simulink model "dft_8_point"  (R2016b)
settings: Solver=VariableStepDiscrete  StartTime=0.0  StopTime=12/fs  RelTol=1e-3  EnableMultiTasking=on
PreLoadFcn:
  | t = 2;
  | b = 14;
  | 
  | fs = 1;
StartFcn:
  | close all;
StopFcn:
  | % create matrices of Re and Im parts over time - inputs
  | xin_re = [xin_0_re xin_1_re xin_2_re xin_3_re xin_4_re xin_5_re xin_6_re xin_7_re];
  | xin_im = [xin_0_im xin_0_im xin_0_im xin_0_im xin_0_im xin_0_im xin_0_im xin_0_im];
  | 
  | % create matrices of Re and Im parts over time - outputs
  | X_re = [X0_re X1_re X2_re X3_re X4_re X5_re X6_re X7_re];
  | X_im = [X0_im X1_im X2_im X3_im X4_im X5_im X6_im X7_im];
  | 
  | % create vectors of Magnitudes and Angles over time
  | X_mag = [X0_mag X1_mag X2_mag X3_mag X4_mag X5_mag X6_mag X7_mag];
  | X_ang = [X0_ang X1_ang X2_ang X3_ang X4_ang X5_ang X6_ang X7_ang];
  | 
  | 
  | figure(1)
  | hold off
  | plot([0:1:7],xin_re(end,:),'r-o','MarkerFaceColor','r');
  | hold on
  | plot([0:1:7],xin_im(end,:),'b-o','MarkerFaceColor','b');
  | xlabel('Samples');
  | ylabel('Magnitude');
  | title('Input to DFT');
  | legend('Real','Imaginary','Location','EastOutside')
  | grid on;
  | 
  | set(1,'Name','Input to DFT','NumberTitle','off');
  | % setStandardFigSize(1);
  | 
  | figure(2)
  | hold off
  | plot([0:1:7],X_mag(end,:),'k-o','MarkerFaceColor','b');
  | hold on
  | xlabel('Frequency Bin');
  | ylabel('Magnitude');
  | grid on;
  | title('Magnitude DFT Plot');
  | 
  | set(2,'Name','Output of DFT','NumberTitle','off');
  | % setStandardFigSize(2);
libraries: xbsIndex_r4 x955
(part 8 of 8)

== system dft_8_point/cplx_add45 ==
  a_im : Inport
  b_im : Inport  Port=2
  a_re : Inport  Port=3
  b_re : Inport  Port=4
  AddSub13 : xbsIndex_r4/AddSub  mode=Addition  use_carryin=off  use_carryout=off  en=off  latency=0  precision=User Defined  arith_type="Signed  (2's comp)"  n_bits=t+b  bin_pt=b  quantization=Truncate  overflow=Wrap  use_behavioral_HDL=off  hw_selection=Fabric  pipelined=off  dbl_ovrd=off  block_type=addsub
  AddSub6 : xbsIndex_r4/AddSub  mode=Addition  use_carryin=off  use_carryout=off  en=off  latency=0  precision=User Defined  arith_type="Signed  (2's comp)"  n_bits=t+b  bin_pt=b  quantization=Truncate  overflow=Wrap  use_behavioral_HDL=off  hw_selection=Fabric  pipelined=off  dbl_ovrd=off  block_type=addsub
  im : Outport
  re : Outport  Port=2
  wires:
  a_im/1 -> AddSub6/1
  AddSub6/1 -> im/1
  b_im/1 -> AddSub6/2
  a_re/1 -> AddSub13/1
  AddSub13/1 -> re/1
  b_re/1 -> AddSub13/2

== system dft_8_point/cplx_add46 ==
  a_im : Inport
  b_im : Inport  Port=2
  a_re : Inport  Port=3
  b_re : Inport  Port=4
  AddSub13 : xbsIndex_r4/AddSub  mode=Addition  use_carryin=off  use_carryout=off  en=off  latency=0  precision=User Defined  arith_type="Signed  (2's comp)"  n_bits=t+b  bin_pt=b  quantization=Truncate  overflow=Wrap  use_behavioral_HDL=off  hw_selection=Fabric  pipelined=off  dbl_ovrd=off  block_type=addsub
  AddSub6 : xbsIndex_r4/AddSub  mode=Addition  use_carryin=off  use_carryout=off  en=off  latency=0  precision=User Defined  arith_type="Signed  (2's comp)"  n_bits=t+b  bin_pt=b  quantization=Truncate  overflow=Wrap  use_behavioral_HDL=off  hw_selection=Fabric  pipelined=off  dbl_ovrd=off  block_type=addsub
  im : Outport
  re : Outport  Port=2
  wires:
  a_im/1 -> AddSub6/1
  AddSub6/1 -> im/1
  b_im/1 -> AddSub6/2
  a_re/1 -> AddSub13/1
  AddSub13/1 -> re/1
  b_re/1 -> AddSub13/2

== system dft_8_point/cplx_add47 ==
  a_im : Inport
  b_im : Inport  Port=2
  a_re : Inport  Port=3
  b_re : Inport  Port=4
  AddSub13 : xbsIndex_r4/AddSub  mode=Addition  use_carryin=off  use_carryout=off  en=off  latency=0  precision=User Defined  arith_type="Signed  (2's comp)"  n_bits=t+b  bin_pt=b  quantization=Truncate  overflow=Wrap  use_behavioral_HDL=off  hw_selection=Fabric  pipelined=off  dbl_ovrd=off  block_type=addsub
  AddSub6 : xbsIndex_r4/AddSub  mode=Addition  use_carryin=off  use_carryout=off  en=off  latency=0  precision=User Defined  arith_type="Signed  (2's comp)"  n_bits=t+b  bin_pt=b  quantization=Truncate  overflow=Wrap  use_behavioral_HDL=off  hw_selection=Fabric  pipelined=off  dbl_ovrd=off  block_type=addsub
  im : Outport
  re : Outport  Port=2
  wires:
  a_im/1 -> AddSub6/1
  AddSub6/1 -> im/1
  b_im/1 -> AddSub6/2
  a_re/1 -> AddSub13/1
  AddSub13/1 -> re/1
  b_re/1 -> AddSub13/2

== system dft_8_point/cplx_add48 ==
  a_im : Inport
  b_im : Inport  Port=2
  a_re : Inport  Port=3
  b_re : Inport  Port=4
  AddSub13 : xbsIndex_r4/AddSub  mode=Addition  use_carryin=off  use_carryout=off  en=off  latency=0  precision=User Defined  arith_type="Signed  (2's comp)"  n_bits=t+b  bin_pt=b  quantization=Truncate  overflow=Wrap  use_behavioral_HDL=off  hw_selection=Fabric  pipelined=off  dbl_ovrd=off  block_type=addsub
  AddSub6 : xbsIndex_r4/AddSub  mode=Addition  use_carryin=off  use_carryout=off  en=off  latency=0  precision=User Defined  arith_type="Signed  (2's comp)"  n_bits=t+b  bin_pt=b  quantization=Truncate  overflow=Wrap  use_behavioral_HDL=off  hw_selection=Fabric  pipelined=off  dbl_ovrd=off  block_type=addsub
  im : Outport
  re : Outport  Port=2
  wires:
  a_im/1 -> AddSub6/1
  AddSub6/1 -> im/1
  b_im/1 -> AddSub6/2
  a_re/1 -> AddSub13/1
  AddSub13/1 -> re/1
  b_re/1 -> AddSub13/2

== system dft_8_point/cplx_add49 ==
  a_im : Inport
  b_im : Inport  Port=2
  a_re : Inport  Port=3
  b_re : Inport  Port=4
  AddSub13 : xbsIndex_r4/AddSub  mode=Addition  use_carryin=off  use_carryout=off  en=off  latency=0  precision=User Defined  arith_type="Signed  (2's comp)"  n_bits=t+b  bin_pt=b  quantization=Truncate  overflow=Wrap  use_behavioral_HDL=off  hw_selection=Fabric  pipelined=off  dbl_ovrd=off  block_type=addsub
  AddSub6 : xbsIndex_r4/AddSub  mode=Addition  use_carryin=off  use_carryout=off  en=off  latency=0  precision=User Defined  arith_type="Signed  (2's comp)"  n_bits=t+b  bin_pt=b  quantization=Truncate  overflow=Wrap  use_behavioral_HDL=off  hw_selection=Fabric  pipelined=off  dbl_ovrd=off  block_type=addsub
  im : Outport
  re : Outport  Port=2
  wires:
  a_im/1 -> AddSub6/1
  AddSub6/1 -> im/1
  b_im/1 -> AddSub6/2
  a_re/1 -> AddSub13/1
  AddSub13/1 -> re/1
  b_re/1 -> AddSub13/2

== system dft_8_point/cplx_add5 ==
  a_im : Inport
  b_im : Inport  Port=2
  a_re : Inport  Port=3
  b_re : Inport  Port=4
  AddSub13 : xbsIndex_r4/AddSub  mode=Addition  use_carryin=off  use_carryout=off  en=off  latency=0  precision=User Defined  arith_type="Signed  (2's comp)"  n_bits=t+b  bin_pt=b  quantization=Truncate  overflow=Wrap  use_behavioral_HDL=off  hw_selection=Fabric  pipelined=off  dbl_ovrd=off  block_type=addsub
  AddSub6 : xbsIndex_r4/AddSub  mode=Addition  use_carryin=off  use_carryout=off  en=off  latency=0  precision=User Defined  arith_type="Signed  (2's comp)"  n_bits=t+b  bin_pt=b  quantization=Truncate  overflow=Wrap  use_behavioral_HDL=off  hw_selection=Fabric  pipelined=off  dbl_ovrd=off  block_type=addsub
  im : Outport
  re : Outport  Port=2
  wires:
  a_im/1 -> AddSub6/1
  AddSub6/1 -> im/1
  b_im/1 -> AddSub6/2
  a_re/1 -> AddSub13/1
  AddSub13/1 -> re/1
  b_re/1 -> AddSub13/2

== system dft_8_point/cplx_add50 ==
  a_im : Inport
  b_im : Inport  Port=2
  a_re : Inport  Port=3
  b_re : Inport  Port=4
  AddSub13 : xbsIndex_r4/AddSub  mode=Addition  use_carryin=off  use_carryout=off  en=off  latency=0  precision=User Defined  arith_type="Signed  (2's comp)"  n_bits=t+b  bin_pt=b  quantization=Truncate  overflow=Wrap  use_behavioral_HDL=off  hw_selection=Fabric  pipelined=off  dbl_ovrd=off  block_type=addsub
  AddSub6 : xbsIndex_r4/AddSub  mode=Addition  use_carryin=off  use_carryout=off  en=off  latency=0  precision=User Defined  arith_type="Signed  (2's comp)"  n_bits=t+b  bin_pt=b  quantization=Truncate  overflow=Wrap  use_behavioral_HDL=off  hw_selection=Fabric  pipelined=off  dbl_ovrd=off  block_type=addsub
  im : Outport
  re : Outport  Port=2
  wires:
  a_im/1 -> AddSub6/1
  AddSub6/1 -> im/1
  b_im/1 -> AddSub6/2
  a_re/1 -> AddSub13/1
  AddSub13/1 -> re/1
  b_re/1 -> AddSub13/2

== system dft_8_point/cplx_add51 ==
  a_im : Inport
  b_im : Inport  Port=2
  a_re : Inport  Port=3
  b_re : Inport  Port=4
  AddSub13 : xbsIndex_r4/AddSub  mode=Addition  use_carryin=off  use_carryout=off  en=off  latency=0  precision=User Defined  arith_type="Signed  (2's comp)"  n_bits=t+b  bin_pt=b  quantization=Truncate  overflow=Wrap  use_behavioral_HDL=off  hw_selection=Fabric  pipelined=off  dbl_ovrd=off  block_type=addsub
  AddSub6 : xbsIndex_r4/AddSub  mode=Addition  use_carryin=off  use_carryout=off  en=off  latency=0  precision=User Defined  arith_type="Signed  (2's comp)"  n_bits=t+b  bin_pt=b  quantization=Truncate  overflow=Wrap  use_behavioral_HDL=off  hw_selection=Fabric  pipelined=off  dbl_ovrd=off  block_type=addsub
  im : Outport
  re : Outport  Port=2
  wires:
  a_im/1 -> AddSub6/1
  AddSub6/1 -> im/1
  b_im/1 -> AddSub6/2
  a_re/1 -> AddSub13/1
  AddSub13/1 -> re/1
  b_re/1 -> AddSub13/2

== system dft_8_point/cplx_add52 ==
  a_im : Inport
  b_im : Inport  Port=2
  a_re : Inport  Port=3
  b_re : Inport  Port=4
  AddSub13 : xbsIndex_r4/AddSub  mode=Addition  use_carryin=off  use_carryout=off  en=off  latency=0  precision=User Defined  arith_type="Signed  (2's comp)"  n_bits=t+b  bin_pt=b  quantization=Truncate  overflow=Wrap  use_behavioral_HDL=off  hw_selection=Fabric  pipelined=off  dbl_ovrd=off  block_type=addsub
  AddSub6 : xbsIndex_r4/AddSub  mode=Addition  use_carryin=off  use_carryout=off  en=off  latency=0  precision=User Defined  arith_type="Signed  (2's comp)"  n_bits=t+b  bin_pt=b  quantization=Truncate  overflow=Wrap  use_behavioral_HDL=off  hw_selection=Fabric  pipelined=off  dbl_ovrd=off  block_type=addsub
  im : Outport
  re : Outport  Port=2
  wires:
  a_im/1 -> AddSub6/1
  AddSub6/1 -> im/1
  b_im/1 -> AddSub6/2
  a_re/1 -> AddSub13/1
  AddSub13/1 -> re/1
  b_re/1 -> AddSub13/2

== system dft_8_point/cplx_add53 ==
  a_im : Inport
  b_im : Inport  Port=2
  a_re : Inport  Port=3
  b_re : Inport  Port=4
  AddSub13 : xbsIndex_r4/AddSub  mode=Addition  use_carryin=off  use_carryout=off  en=off  latency=0  precision=User Defined  arith_type="Signed  (2's comp)"  n_bits=t+b  bin_pt=b  quantization=Truncate  overflow=Wrap  use_behavioral_HDL=off  hw_selection=Fabric  pipelined=off  dbl_ovrd=off  block_type=addsub
  AddSub6 : xbsIndex_r4/AddSub  mode=Addition  use_carryin=off  use_carryout=off  en=off  latency=0  precision=User Defined  arith_type="Signed  (2's comp)"  n_bits=t+b  bin_pt=b  quantization=Truncate  overflow=Wrap  use_behavioral_HDL=off  hw_selection=Fabric  pipelined=off  dbl_ovrd=off  block_type=addsub
  im : Outport
  re : Outport  Port=2
  wires:
  a_im/1 -> AddSub6/1
  AddSub6/1 -> im/1
  b_im/1 -> AddSub6/2
  a_re/1 -> AddSub13/1
  AddSub13/1 -> re/1
  b_re/1 -> AddSub13/2

== system dft_8_point/cplx_add54 ==
  a_im : Inport
  b_im : Inport  Port=2
  a_re : Inport  Port=3
  b_re : Inport  Port=4
  AddSub13 : xbsIndex_r4/AddSub  mode=Addition  use_carryin=off  use_carryout=off  en=off  latency=0  precision=User Defined  arith_type="Signed  (2's comp)"  n_bits=t+b  bin_pt=b  quantization=Truncate  overflow=Wrap  use_behavioral_HDL=off  hw_selection=Fabric  pipelined=off  dbl_ovrd=off  block_type=addsub
  AddSub6 : xbsIndex_r4/AddSub  mode=Addition  use_carryin=off  use_carryout=off  en=off  latency=0  precision=User Defined  arith_type="Signed  (2's comp)"  n_bits=t+b  bin_pt=b  quantization=Truncate  overflow=Wrap  use_behavioral_HDL=off  hw_selection=Fabric  pipelined=off  dbl_ovrd=off  block_type=addsub
  im : Outport
  re : Outport  Port=2
  wires:
  a_im/1 -> AddSub6/1
  AddSub6/1 -> im/1
  b_im/1 -> AddSub6/2
  a_re/1 -> AddSub13/1
  AddSub13/1 -> re/1
  b_re/1 -> AddSub13/2

== system dft_8_point/cplx_add55 ==
  a_im : Inport
  b_im : Inport  Port=2
  a_re : Inport  Port=3
  b_re : Inport  Port=4
  AddSub13 : xbsIndex_r4/AddSub  mode=Addition  use_carryin=off  use_carryout=off  en=off  latency=0  precision=User Defined  arith_type="Signed  (2's comp)"  n_bits=t+b  bin_pt=b  quantization=Truncate  overflow=Wrap  use_behavioral_HDL=off  hw_selection=Fabric  pipelined=off  dbl_ovrd=off  block_type=addsub
  AddSub6 : xbsIndex_r4/AddSub  mode=Addition  use_carryin=off  use_carryout=off  en=off  latency=0  precision=User Defined  arith_type="Signed  (2's comp)"  n_bits=t+b  bin_pt=b  quantization=Truncate  overflow=Wrap  use_behavioral_HDL=off  hw_selection=Fabric  pipelined=off  dbl_ovrd=off  block_type=addsub
  im : Outport
  re : Outport  Port=2
  wires:
  a_im/1 -> AddSub6/1
  AddSub6/1 -> im/1
  b_im/1 -> AddSub6/2
  a_re/1 -> AddSub13/1
  AddSub13/1 -> re/1
  b_re/1 -> AddSub13/2

== system dft_8_point/cplx_add6 ==
  a_im : Inport
  b_im : Inport  Port=2
  a_re : Inport  Port=3
  b_re : Inport  Port=4
  AddSub13 : xbsIndex_r4/AddSub  mode=Addition  use_carryin=off  use_carryout=off  en=off  latency=0  precision=User Defined  arith_type="Signed  (2's comp)"  n_bits=t+b  bin_pt=b  quantization=Truncate  overflow=Wrap  use_behavioral_HDL=off  hw_selection=Fabric  pipelined=off  dbl_ovrd=off  block_type=addsub
  AddSub6 : xbsIndex_r4/AddSub  mode=Addition  use_carryin=off  use_carryout=off  en=off  latency=0  precision=User Defined  arith_type="Signed  (2's comp)"  n_bits=t+b  bin_pt=b  quantization=Truncate  overflow=Wrap  use_behavioral_HDL=off  hw_selection=Fabric  pipelined=off  dbl_ovrd=off  block_type=addsub
  im : Outport
  re : Outport  Port=2
  wires:
  a_im/1 -> AddSub6/1
  AddSub6/1 -> im/1
  b_im/1 -> AddSub6/2
  a_re/1 -> AddSub13/1
  AddSub13/1 -> re/1
  b_re/1 -> AddSub13/2

== system dft_8_point/cplx_add7 ==
  a_im : Inport
  b_im : Inport  Port=2
  a_re : Inport  Port=3
  b_re : Inport  Port=4
  AddSub13 : xbsIndex_r4/AddSub  mode=Addition  use_carryin=off  use_carryout=off  en=off  latency=0  precision=User Defined  arith_type="Signed  (2's comp)"  n_bits=t+b  bin_pt=b  quantization=Truncate  overflow=Wrap  use_behavioral_HDL=off  hw_selection=Fabric  pipelined=off  dbl_ovrd=off  block_type=addsub
  AddSub6 : xbsIndex_r4/AddSub  mode=Addition  use_carryin=off  use_carryout=off  en=off  latency=0  precision=User Defined  arith_type="Signed  (2's comp)"  n_bits=t+b  bin_pt=b  quantization=Truncate  overflow=Wrap  use_behavioral_HDL=off  hw_selection=Fabric  pipelined=off  dbl_ovrd=off  block_type=addsub
  im : Outport
  re : Outport  Port=2
  wires:
  a_im/1 -> AddSub6/1
  AddSub6/1 -> im/1
  b_im/1 -> AddSub6/2
  a_re/1 -> AddSub13/1
  AddSub13/1 -> re/1
  b_re/1 -> AddSub13/2

== system dft_8_point/cplx_add8 ==
  a_im : Inport
  b_im : Inport  Port=2
  a_re : Inport  Port=3
  b_re : Inport  Port=4
  AddSub13 : xbsIndex_r4/AddSub  mode=Addition  use_carryin=off  use_carryout=off  en=off  latency=0  precision=User Defined  arith_type="Signed  (2's comp)"  n_bits=t+b  bin_pt=b  quantization=Truncate  overflow=Wrap  use_behavioral_HDL=off  hw_selection=Fabric  pipelined=off  dbl_ovrd=off  block_type=addsub
  AddSub6 : xbsIndex_r4/AddSub  mode=Addition  use_carryin=off  use_carryout=off  en=off  latency=0  precision=User Defined  arith_type="Signed  (2's comp)"  n_bits=t+b  bin_pt=b  quantization=Truncate  overflow=Wrap  use_behavioral_HDL=off  hw_selection=Fabric  pipelined=off  dbl_ovrd=off  block_type=addsub
  im : Outport
  re : Outport  Port=2
  wires:
  a_im/1 -> AddSub6/1
  AddSub6/1 -> im/1
  b_im/1 -> AddSub6/2
  a_re/1 -> AddSub13/1
  AddSub13/1 -> re/1
  b_re/1 -> AddSub13/2

== system dft_8_point/cplx_add9 ==
  a_im : Inport
  b_im : Inport  Port=2
  a_re : Inport  Port=3
  b_re : Inport  Port=4
  AddSub13 : xbsIndex_r4/AddSub  mode=Addition  use_carryin=off  use_carryout=off  en=off  latency=0  precision=User Defined  arith_type="Signed  (2's comp)"  n_bits=t+b  bin_pt=b  quantization=Truncate  overflow=Wrap  use_behavioral_HDL=off  hw_selection=Fabric  pipelined=off  dbl_ovrd=off  block_type=addsub
  AddSub6 : xbsIndex_r4/AddSub  mode=Addition  use_carryin=off  use_carryout=off  en=off  latency=0  precision=User Defined  arith_type="Signed  (2's comp)"  n_bits=t+b  bin_pt=b  quantization=Truncate  overflow=Wrap  use_behavioral_HDL=off  hw_selection=Fabric  pipelined=off  dbl_ovrd=off  block_type=addsub
  im : Outport
  re : Outport  Port=2
  wires:
  a_im/1 -> AddSub6/1
  AddSub6/1 -> im/1
  b_im/1 -> AddSub6/2
  a_re/1 -> AddSub13/1
  AddSub13/1 -> re/1
  b_re/1 -> AddSub13/2

== system dft_8_point/Capture Delay Line Inputs/cplx_split1 ==
  cmplx : Inport
  Reinterpret : xbsIndex_r4/Reinterpret  force_arith_type=on  arith_type="Signed  (2's comp)"  force_bin_pt=on  bin_pt=b  block_type=reinterpret
      settings: infoedit="Changes signal type without altering the binary representation.   You can changed the signal between signed and unsigned, and relocate the binary point.<br><br>Hardware notes: In hardware this block costs nothing.<br><br>Example:  Suppose the input is 6 bits wide, signed, with 2 fractional bits, and the output is forced to unsigned with 0 fractional bits.  Then an input of -2.0 (1110.00 in binary 2's complement) becomes an output of 56 (111000 in binary)."
  Reinterpret1 : xbsIndex_r4/Reinterpret  force_arith_type=on  arith_type="Signed  (2's comp)"  force_bin_pt=on  bin_pt=b  block_type=reinterpret
      settings: infoedit="Changes signal type without altering the binary representation.   You can changed the signal between signed and unsigned, and relocate the binary point.<br><br>Hardware notes: In hardware this block costs nothing.<br><br>Example:  Suppose the input is 6 bits wide, signed, with 2 fractional bits, and the output is forced to unsigned with 0 fractional bits.  Then an input of -2.0 (1110.00 in binary 2's complement) becomes an output of 56 (111000 in binary)."
  x_imaginary : xbsIndex_r4/Slice  nbits=t+b  boolean_output=off  mode=Lower Bit Location + Width  bit1=0  base1=MSB of Input  bit0=0  base0=LSB of Input  dbl_ovrd=off  block_type=slice
  x_real : xbsIndex_r4/Slice  nbits=t+b  boolean_output=off  mode=Upper Bit Location + Width  bit1=0  base1=MSB of Input  bit0=0  base0=LSB of Input  dbl_ovrd=off  block_type=slice
  real : Outport
  imag : Outport  Port=2
  wires:
  cmplx/1 -> x_real/1, x_imaginary/1
  x_real/1 -> Reinterpret/1
  x_imaginary/1 -> Reinterpret1/1
  Reinterpret/1 -> real/1
  Reinterpret1/1 -> imag/1

== system dft_8_point/Capture Delay Line Inputs/cplx_split2 ==
  cmplx : Inport
  Reinterpret : xbsIndex_r4/Reinterpret  force_arith_type=on  arith_type="Signed  (2's comp)"  force_bin_pt=on  bin_pt=b  block_type=reinterpret
      settings: infoedit="Changes signal type without altering the binary representation.   You can changed the signal between signed and unsigned, and relocate the binary point.<br><br>Hardware notes: In hardware this block costs nothing.<br><br>Example:  Suppose the input is 6 bits wide, signed, with 2 fractional bits, and the output is forced to unsigned with 0 fractional bits.  Then an input of -2.0 (1110.00 in binary 2's complement) becomes an output of 56 (111000 in binary)."
  Reinterpret1 : xbsIndex_r4/Reinterpret  force_arith_type=on  arith_type="Signed  (2's comp)"  force_bin_pt=on  bin_pt=b  block_type=reinterpret
      settings: infoedit="Changes signal type without altering the binary representation.   You can changed the signal between signed and unsigned, and relocate the binary point.<br><br>Hardware notes: In hardware this block costs nothing.<br><br>Example:  Suppose the input is 6 bits wide, signed, with 2 fractional bits, and the output is forced to unsigned with 0 fractional bits.  Then an input of -2.0 (1110.00 in binary 2's complement) becomes an output of 56 (111000 in binary)."
  x_imaginary : xbsIndex_r4/Slice  nbits=t+b  boolean_output=off  mode=Lower Bit Location + Width  bit1=0  base1=MSB of Input  bit0=0  base0=LSB of Input  dbl_ovrd=off  block_type=slice
  x_real : xbsIndex_r4/Slice  nbits=t+b  boolean_output=off  mode=Upper Bit Location + Width  bit1=0  base1=MSB of Input  bit0=0  base0=LSB of Input  dbl_ovrd=off  block_type=slice
  real : Outport
  imag : Outport  Port=2
  wires:
  cmplx/1 -> x_real/1, x_imaginary/1
  x_real/1 -> Reinterpret/1
  x_imaginary/1 -> Reinterpret1/1
  Reinterpret/1 -> real/1
  Reinterpret1/1 -> imag/1

== system dft_8_point/Capture Delay Line Inputs/cplx_split3 ==
  cmplx : Inport
  Reinterpret : xbsIndex_r4/Reinterpret  force_arith_type=on  arith_type="Signed  (2's comp)"  force_bin_pt=on  bin_pt=b  block_type=reinterpret
      settings: infoedit="Changes signal type without altering the binary representation.   You can changed the signal between signed and unsigned, and relocate the binary point.<br><br>Hardware notes: In hardware this block costs nothing.<br><br>Example:  Suppose the input is 6 bits wide, signed, with 2 fractional bits, and the output is forced to unsigned with 0 fractional bits.  Then an input of -2.0 (1110.00 in binary 2's complement) becomes an output of 56 (111000 in binary)."
  Reinterpret1 : xbsIndex_r4/Reinterpret  force_arith_type=on  arith_type="Signed  (2's comp)"  force_bin_pt=on  bin_pt=b  block_type=reinterpret
      settings: infoedit="Changes signal type without altering the binary representation.   You can changed the signal between signed and unsigned, and relocate the binary point.<br><br>Hardware notes: In hardware this block costs nothing.<br><br>Example:  Suppose the input is 6 bits wide, signed, with 2 fractional bits, and the output is forced to unsigned with 0 fractional bits.  Then an input of -2.0 (1110.00 in binary 2's complement) becomes an output of 56 (111000 in binary)."
  x_imaginary : xbsIndex_r4/Slice  nbits=t+b  boolean_output=off  mode=Lower Bit Location + Width  bit1=0  base1=MSB of Input  bit0=0  base0=LSB of Input  dbl_ovrd=off  block_type=slice
  x_real : xbsIndex_r4/Slice  nbits=t+b  boolean_output=off  mode=Upper Bit Location + Width  bit1=0  base1=MSB of Input  bit0=0  base0=LSB of Input  dbl_ovrd=off  block_type=slice
  real : Outport
  imag : Outport  Port=2
  wires:
  cmplx/1 -> x_real/1, x_imaginary/1
  x_real/1 -> Reinterpret/1
  x_imaginary/1 -> Reinterpret1/1
  Reinterpret/1 -> real/1
  Reinterpret1/1 -> imag/1

== system dft_8_point/Capture Delay Line Inputs/cplx_split4 ==
  cmplx : Inport
  Reinterpret : xbsIndex_r4/Reinterpret  force_arith_type=on  arith_type="Signed  (2's comp)"  force_bin_pt=on  bin_pt=b  block_type=reinterpret
      settings: infoedit="Changes signal type without altering the binary representation.   You can changed the signal between signed and unsigned, and relocate the binary point.<br><br>Hardware notes: In hardware this block costs nothing.<br><br>Example:  Suppose the input is 6 bits wide, signed, with 2 fractional bits, and the output is forced to unsigned with 0 fractional bits.  Then an input of -2.0 (1110.00 in binary 2's complement) becomes an output of 56 (111000 in binary)."
  Reinterpret1 : xbsIndex_r4/Reinterpret  force_arith_type=on  arith_type="Signed  (2's comp)"  force_bin_pt=on  bin_pt=b  block_type=reinterpret
      settings: infoedit="Changes signal type without altering the binary representation.   You can changed the signal between signed and unsigned, and relocate the binary point.<br><br>Hardware notes: In hardware this block costs nothing.<br><br>Example:  Suppose the input is 6 bits wide, signed, with 2 fractional bits, and the output is forced to unsigned with 0 fractional bits.  Then an input of -2.0 (1110.00 in binary 2's complement) becomes an output of 56 (111000 in binary)."
  x_imaginary : xbsIndex_r4/Slice  nbits=t+b  boolean_output=off  mode=Lower Bit Location + Width  bit1=0  base1=MSB of Input  bit0=0  base0=LSB of Input  dbl_ovrd=off  block_type=slice
  x_real : xbsIndex_r4/Slice  nbits=t+b  boolean_output=off  mode=Upper Bit Location + Width  bit1=0  base1=MSB of Input  bit0=0  base0=LSB of Input  dbl_ovrd=off  block_type=slice
  real : Outport
  imag : Outport  Port=2
  wires:
  cmplx/1 -> x_real/1, x_imaginary/1
  x_real/1 -> Reinterpret/1
  x_imaginary/1 -> Reinterpret1/1
  Reinterpret/1 -> real/1
  Reinterpret1/1 -> imag/1

== system dft_8_point/Capture Delay Line Inputs/cplx_split5 ==
  cmplx : Inport
  Reinterpret : xbsIndex_r4/Reinterpret  force_arith_type=on  arith_type="Signed  (2's comp)"  force_bin_pt=on  bin_pt=b  block_type=reinterpret
      settings: infoedit="Changes signal type without altering the binary representation.   You can changed the signal between signed and unsigned, and relocate the binary point.<br><br>Hardware notes: In hardware this block costs nothing.<br><br>Example:  Suppose the input is 6 bits wide, signed, with 2 fractional bits, and the output is forced to unsigned with 0 fractional bits.  Then an input of -2.0 (1110.00 in binary 2's complement) becomes an output of 56 (111000 in binary)."
  Reinterpret1 : xbsIndex_r4/Reinterpret  force_arith_type=on  arith_type="Signed  (2's comp)"  force_bin_pt=on  bin_pt=b  block_type=reinterpret
      settings: infoedit="Changes signal type without altering the binary representation.   You can changed the signal between signed and unsigned, and relocate the binary point.<br><br>Hardware notes: In hardware this block costs nothing.<br><br>Example:  Suppose the input is 6 bits wide, signed, with 2 fractional bits, and the output is forced to unsigned with 0 fractional bits.  Then an input of -2.0 (1110.00 in binary 2's complement) becomes an output of 56 (111000 in binary)."
  x_imaginary : xbsIndex_r4/Slice  nbits=t+b  boolean_output=off  mode=Lower Bit Location + Width  bit1=0  base1=MSB of Input  bit0=0  base0=LSB of Input  dbl_ovrd=off  block_type=slice
  x_real : xbsIndex_r4/Slice  nbits=t+b  boolean_output=off  mode=Upper Bit Location + Width  bit1=0  base1=MSB of Input  bit0=0  base0=LSB of Input  dbl_ovrd=off  block_type=slice
  real : Outport
  imag : Outport  Port=2
  wires:
  cmplx/1 -> x_real/1, x_imaginary/1
  x_real/1 -> Reinterpret/1
  x_imaginary/1 -> Reinterpret1/1
  Reinterpret/1 -> real/1
  Reinterpret1/1 -> imag/1

== system dft_8_point/Capture Delay Line Inputs/cplx_split6 ==
  cmplx : Inport
  Reinterpret : xbsIndex_r4/Reinterpret  force_arith_type=on  arith_type="Signed  (2's comp)"  force_bin_pt=on  bin_pt=b  block_type=reinterpret
      settings: infoedit="Changes signal type without altering the binary representation.   You can changed the signal between signed and unsigned, and relocate the binary point.<br><br>Hardware notes: In hardware this block costs nothing.<br><br>Example:  Suppose the input is 6 bits wide, signed, with 2 fractional bits, and the output is forced to unsigned with 0 fractional bits.  Then an input of -2.0 (1110.00 in binary 2's complement) becomes an output of 56 (111000 in binary)."
  Reinterpret1 : xbsIndex_r4/Reinterpret  force_arith_type=on  arith_type="Signed  (2's comp)"  force_bin_pt=on  bin_pt=b  block_type=reinterpret
      settings: infoedit="Changes signal type without altering the binary representation.   You can changed the signal between signed and unsigned, and relocate the binary point.<br><br>Hardware notes: In hardware this block costs nothing.<br><br>Example:  Suppose the input is 6 bits wide, signed, with 2 fractional bits, and the output is forced to unsigned with 0 fractional bits.  Then an input of -2.0 (1110.00 in binary 2's complement) becomes an output of 56 (111000 in binary)."
  x_imaginary : xbsIndex_r4/Slice  nbits=t+b  boolean_output=off  mode=Lower Bit Location + Width  bit1=0  base1=MSB of Input  bit0=0  base0=LSB of Input  dbl_ovrd=off  block_type=slice
  x_real : xbsIndex_r4/Slice  nbits=t+b  boolean_output=off  mode=Upper Bit Location + Width  bit1=0  base1=MSB of Input  bit0=0  base0=LSB of Input  dbl_ovrd=off  block_type=slice
  real : Outport
  imag : Outport  Port=2
  wires:
  cmplx/1 -> x_real/1, x_imaginary/1
  x_real/1 -> Reinterpret/1
  x_imaginary/1 -> Reinterpret1/1
  Reinterpret/1 -> real/1
  Reinterpret1/1 -> imag/1

== system dft_8_point/Capture Delay Line Inputs/cplx_split7 ==
  cmplx : Inport
  Reinterpret : xbsIndex_r4/Reinterpret  force_arith_type=on  arith_type="Signed  (2's comp)"  force_bin_pt=on  bin_pt=b  block_type=reinterpret
      settings: infoedit="Changes signal type without altering the binary representation.   You can changed the signal between signed and unsigned, and relocate the binary point.<br><br>Hardware notes: In hardware this block costs nothing.<br><br>Example:  Suppose the input is 6 bits wide, signed, with 2 fractional bits, and the output is forced to unsigned with 0 fractional bits.  Then an input of -2.0 (1110.00 in binary 2's complement) becomes an output of 56 (111000 in binary)."
  Reinterpret1 : xbsIndex_r4/Reinterpret  force_arith_type=on  arith_type="Signed  (2's comp)"  force_bin_pt=on  bin_pt=b  block_type=reinterpret
      settings: infoedit="Changes signal type without altering the binary representation.   You can changed the signal between signed and unsigned, and relocate the binary point.<br><br>Hardware notes: In hardware this block costs nothing.<br><br>Example:  Suppose the input is 6 bits wide, signed, with 2 fractional bits, and the output is forced to unsigned with 0 fractional bits.  Then an input of -2.0 (1110.00 in binary 2's complement) becomes an output of 56 (111000 in binary)."
  x_imaginary : xbsIndex_r4/Slice  nbits=t+b  boolean_output=off  mode=Lower Bit Location + Width  bit1=0  base1=MSB of Input  bit0=0  base0=LSB of Input  dbl_ovrd=off  block_type=slice
  x_real : xbsIndex_r4/Slice  nbits=t+b  boolean_output=off  mode=Upper Bit Location + Width  bit1=0  base1=MSB of Input  bit0=0  base0=LSB of Input  dbl_ovrd=off  block_type=slice
  real : Outport
  imag : Outport  Port=2
  wires:
  cmplx/1 -> x_real/1, x_imaginary/1
  x_real/1 -> Reinterpret/1
  x_imaginary/1 -> Reinterpret1/1
  Reinterpret/1 -> real/1
  Reinterpret1/1 -> imag/1

== system dft_8_point/Capture Delay Line Inputs/cplx_split8 ==
  cmplx : Inport
  Reinterpret : xbsIndex_r4/Reinterpret  force_arith_type=on  arith_type="Signed  (2's comp)"  force_bin_pt=on  bin_pt=b  block_type=reinterpret
      settings: infoedit="Changes signal type without altering the binary representation.   You can changed the signal between signed and unsigned, and relocate the binary point.<br><br>Hardware notes: In hardware this block costs nothing.<br><br>Example:  Suppose the input is 6 bits wide, signed, with 2 fractional bits, and the output is forced to unsigned with 0 fractional bits.  Then an input of -2.0 (1110.00 in binary 2's complement) becomes an output of 56 (111000 in binary)."
  Reinterpret1 : xbsIndex_r4/Reinterpret  force_arith_type=on  arith_type="Signed  (2's comp)"  force_bin_pt=on  bin_pt=b  block_type=reinterpret
      settings: infoedit="Changes signal type without altering the binary representation.   You can changed the signal between signed and unsigned, and relocate the binary point.<br><br>Hardware notes: In hardware this block costs nothing.<br><br>Example:  Suppose the input is 6 bits wide, signed, with 2 fractional bits, and the output is forced to unsigned with 0 fractional bits.  Then an input of -2.0 (1110.00 in binary 2's complement) becomes an output of 56 (111000 in binary)."
  x_imaginary : xbsIndex_r4/Slice  nbits=t+b  boolean_output=off  mode=Lower Bit Location + Width  bit1=0  base1=MSB of Input  bit0=0  base0=LSB of Input  dbl_ovrd=off  block_type=slice
  x_real : xbsIndex_r4/Slice  nbits=t+b  boolean_output=off  mode=Upper Bit Location + Width  bit1=0  base1=MSB of Input  bit0=0  base0=LSB of Input  dbl_ovrd=off  block_type=slice
  real : Outport
  imag : Outport  Port=2
  wires:
  cmplx/1 -> x_real/1, x_imaginary/1
  x_real/1 -> Reinterpret/1
  x_imaginary/1 -> Reinterpret1/1
  Reinterpret/1 -> real/1
  Reinterpret1/1 -> imag/1
